simulink model "model_difference_equation"  (R2020b)
settings: Solver=VariableStepAuto  StartTime=0.0  StopTime=10.0  RelTol=1e-3
settings Model: Creator=Training  LastModifiedBy=Training

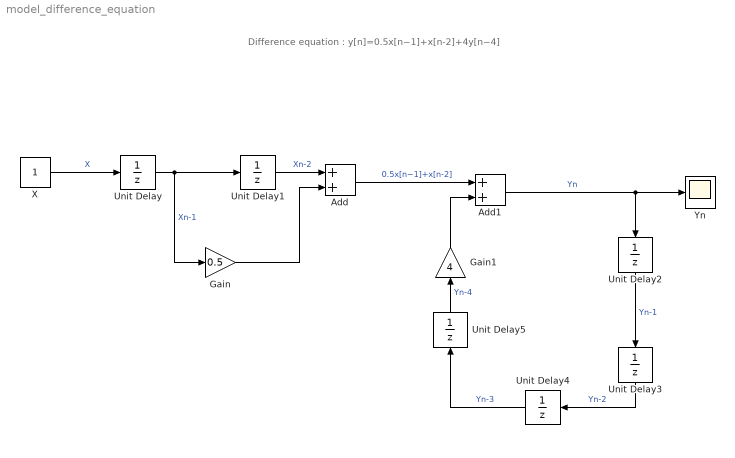
== system model_difference_equation ==
  note: Difference equation : y[n]=0.5x[n−1]+x[n-2]+4y[n−4]
  Add : Sum
  Add1 : Sum
  Gain : Gain  Gain=0.5
  Gain1 : Gain  Gain=4
  Unit Delay : UnitDelay  HasFrameUpgradeWarning=on
  Unit Delay{1..5} (5 alike) : UnitDelay  SampleTime=-1  HasFrameUpgradeWarning=on
  X : Constant
  Yn : Scope
  wires:
  X/1 -> Unit Delay/1  "X"
  Add1/1 -> Unit Delay2/1, Yn/1  "Yn"
  Unit Delay/1 -> Gain/1, Unit Delay1/1  "Xn-1"
  Unit Delay1/1 -> Add/1  "Xn-2"
  Gain/1 -> Add/2
  Unit Delay2/1 -> Unit Delay3/1  "Yn-1"
  Unit Delay3/1 -> Unit Delay4/1  "Yn-2"
  Unit Delay4/1 -> Unit Delay5/1  "Yn-3"
  Add/1 -> Add1/1  "0.5x[n−1]+x[n-2]"
  Unit Delay5/1 -> Gain1/1  "Yn-4"
  Gain1/1 -> Add1/2
